simulink model "precom_dyn_2"  (Simulink 8.7)
settings: Solver=ode45  StartTime=0.0  StopTime=7  FixedStep=.001  RelTol=1e-3
values from neighbouring files (symbols this model uses):
  G = k*(s+c)/(s+a)/(s+b)/(s+b)    [tracer.m]
undefined symbols (not defined in the file or in its folder): A, B, C, F1, Gm, K1
libraries: cstblocks x3
settings Model: Creator=user  LastModifiedBy=NAD
settings DataIOCC: SignalLoggingSaveFormat=ModelDataLogs
settings OptimizationCC: BooleanDataType=off  InitFltsAndDblsToZero=on
settings DebuggingCC: SaveWithParameterizedLinksMsg=none  SignalResolutionControl=TryResolveAllWithWarning  MultiTaskDSMMsg=warning  MultiTaskCondExecSysMsg=none  FcnCallInpInsideContextMsg=UseLocalSettings
settings HardwareCC: TargetBitPerPointer=64  TargetLongLongMode=on  TargetIntDivRoundTo=Zero  TargetEndianess=LittleEndian  TargetWordSize=64  TargetHWDeviceType=MATLAB Host  ProdEqTarget=off
settings GRTTargetCC: TargetFcnLib=ansi_tfl_tmw.mat  CombineOutputUpdateFcns=off  GRTInterface=on

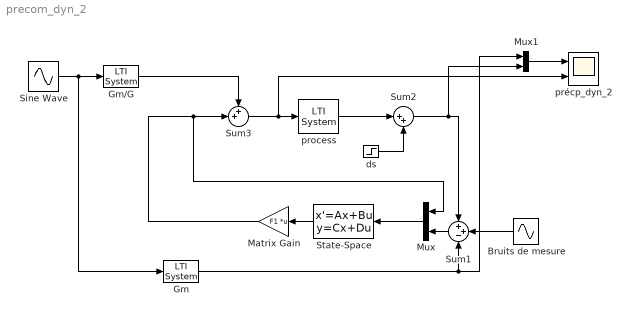
== system precom_dyn_2 ==
  Bruits de mesure : Sin  Frequency=200  SampleTime=0
  Gm : cstblocks/LTI System  sys=Gm  IC=[]
  Gm/G : cstblocks/LTI System  sys=Gm/G  IC=[]
  Matrix Gain : Gain  Gain=F1  Multiplication=Matrix(K*u)  SaturateOnIntegerOverflow=on  OutDataTypeStr=Inherit: Same as input  ParamDataTypeStr=Inherit: Same as input
  Mux : Mux  Inputs=2
  Mux1 : Mux  Inputs=2
  Sine Wave : Sin  SampleTime=0
  State-Space : StateSpace  A=A-K1*C  B=[B K1]  C=eye(3)  D=zeros(3,2)  X0=0
  Sum1 : Sum  Inputs=++-  SaturateOnIntegerOverflow=on  InputSameDT=on  OutDataTypeStr=Inherit: Same as first input
  Sum2 : Sum  Inputs=|++  SaturateOnIntegerOverflow=on  InputSameDT=on  OutDataTypeStr=Inherit: Same as first input
  Sum3 : Sum  Inputs=++|  SaturateOnIntegerOverflow=on  InputSameDT=on  OutDataTypeStr=Inherit: Same as first input
  ds : Step  Time=3  SampleTime=0
  process : cstblocks/LTI System  sys=G  IC=[]
  précp_dyn_2 : Scope  NumInputPorts=2
  wires:
  Mux/1 -> State-Space/1
  State-Space/1 -> Matrix Gain/1
  Matrix Gain/1 -> Sum3/2, Mux/1
  Sine Wave/1 -> Gm/G/1, Gm/1
  Mux1/1 -> précp_dyn_2/1
  process/1 -> Sum2/1
  Sum2/1 -> Mux1/2, Sum1/1
  ds/1 -> Sum2/2
  Sum1/1 -> Mux/2
  Gm/1 -> Mux1/1, Sum1/3
  Gm/G/1 -> Sum3/1
  Sum3/1 -> process/1, précp_dyn_2/2
  Bruits de mesure/1 -> Sum1/2
